simulink model "uloha4"  (R2016b)
settings: Solver=VariableStepAuto  StartTime=0.0  StopTime=10.0  RelTol=1e-3
settings Model: Creator=Milan  LastModifiedBy=Milan

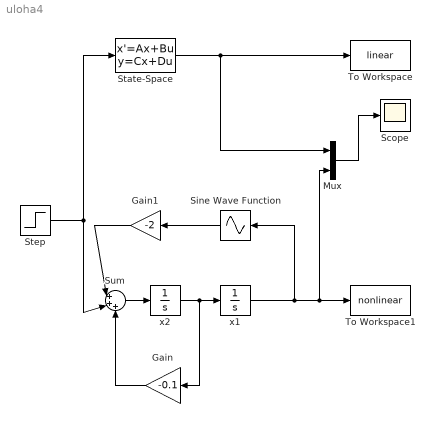
== system uloha4 ==
  Gain : Gain  Gain=-0.1
  Gain1 : Gain  Gain=-2
  Mux : Mux  Inputs=2
  Scope : Scope
  Sine Wave Function : Sin  TimeSource=Use external signal  SampleTime=0
  State-Space : StateSpace  A=[0 1; 0 -0.1]  B=[0; 1]  C=[1 0]  D=0  X0=0
  Step : Step  SampleTime=0
  Sum : Sum  Inputs=|+++
  To Workspace : ToWorkspace  VariableName=linear  SaveFormat=Timeseries  SampleTime=-1
  To Workspace1 : ToWorkspace  VariableName=nonlinear  SaveFormat=Timeseries  SampleTime=-1
  x1 : Integrator
  x2 : Integrator
  wires:
  Step/1 -> Sum/2, State-Space/1
  State-Space/1 -> Mux/1, To Workspace/1
  x2/1 -> Gain/1, x1/1
  Sum/1 -> x2/1
  Gain/1 -> Sum/3
  x1/1 -> Sine Wave Function/1, Mux/2, To Workspace1/1
  Sine Wave Function/1 -> Gain1/1
  Gain1/1 -> Sum/1
  Mux/1 -> Scope/1
